simulink model "TC_SIM_FAST"  (R2025b)
settings: Solver=VariableStepAuto  StartTime=0.0  StopTime=10  RelTol=1e-6
values from neighbouring files (symbols this model uses):
  A = 1    [PARAMS.m]    (also in PARAMS_IDEAL_LAUNCH_TABLE.m; PID_TUNER.m)
  C = 16.56    [PARAMS.m]    (also in PARAMS_IDEAL_LAUNCH_TABLE.m; PID_TUNER.m; r20_18_drive_brake_processing_aaron_comparison.m = -1.75)
  Cd = 1    [PARAMS.m]    (also in PARAMS_IDEAL_LAUNCH_TABLE.m; PID_TUNER.m)
  cg_f = 0.734568    [PARAMS.m]    (also in PARAMS_IDEAL_LAUNCH_TABLE.m; PID_TUNER.m)
  Cl = 3.8    [PARAMS.m]    (also in PARAMS_IDEAL_LAUNCH_TABLE.m; PID_TUNER.m)
  Cp = 0.53    [PARAMS.m]    (also in PARAMS_IDEAL_LAUNCH_TABLE.m; PID_TUNER.m)
  D = 0    [PID_TUNER.m]
  Drive_Train = 0.89    [PARAMS.m]    (also in PARAMS_IDEAL_LAUNCH_TABLE.m; PID_TUNER.m)
  End_Blend = 8.0    (= 8)    [PARAMS.m]    (also in PARAMS_IDEAL_LAUNCH_TABLE.m; PID_TUNER.m)
  fd = 4.5    [PARAMS.m]    (also in PARAMS_IDEAL_LAUNCH_TABLE.m; PID_TUNER.m)
  gravity = 9.80665    [PARAMS.m]    (also in PARAMS_IDEAL_LAUNCH_TABLE.m; PID_TUNER.m)
  Grip_Fact = 1.0    (= 1)    [PARAMS.m]    (also in PARAMS_IDEAL_LAUNCH_TABLE.m; PID_TUNER.m)
  Grip_Influence = 1.2    [PARAMS.m]    (also in PARAMS_IDEAL_LAUNCH_TABLE.m; PID_TUNER.m)
  h_cg = 0.25273    [PARAMS.m]    (also in PARAMS_IDEAL_LAUNCH_TABLE.m; PID_TUNER.m)
  J_Motor = 0.34661    [PARAMS.m]    (also in PARAMS_IDEAL_LAUNCH_TABLE.m; PID_TUNER.m)
  J_Wheel = 0.16490    (= 0.1649)    [PARAMS.m]    (also in PARAMS_IDEAL_LAUNCH_TABLE.m; PID_TUNER.m)
  K = 5105.49    [PARAMS.m]    (also in PARAMS_IDEAL_LAUNCH_TABLE.m; PID_TUNER.m)
  Mv = 285.763    [PARAMS.m]    (also in PARAMS_IDEAL_LAUNCH_TABLE.m; PID_TUNER.m)
  r = 0.203    [PARAMS.m]    (also in PARAMS_IDEAL_LAUNCH_TABLE.m; PID_TUNER.m)
  rho = 1.225    [PARAMS.m]    (also in PARAMS_IDEAL_LAUNCH_TABLE.m; PID_TUNER.m)
  Slip_Target = 0.13    [PARAMS.m]    (also in PARAMS_IDEAL_LAUNCH_TABLE.m; PID_TUNER.m)
  Start_Blend = 3.0    (= 3)    [PARAMS.m]    (also in PARAMS_IDEAL_LAUNCH_TABLE.m; PID_TUNER.m)
  tau_motor = 0.03    [PARAMS.m]    (also in PARAMS_IDEAL_LAUNCH_TABLE.m; PID_TUNER.m = 0.02)
  Throttle_pts = double(launchCmd)/1000    [PARAMS.m]    (also in PARAMS_IDEAL_LAUNCH_TABLE.m = double(launchCmd)/1000.0; PID_TUNER.m = [0.000, 0.364, 0.600, 0.830, 0.903, 0.920, 0.917, 0.903, 0.9; THROTTLE_LOOKUP_GENERATOR.m = [1.000, 1.000, 1.000, 1.000, 1.000, 1.000, 1.000, 1.000, 1.0)
  Time_pts = double(launchTimeMs)/1000    [PARAMS.m]    (also in PARAMS_IDEAL_LAUNCH_TABLE.m = double(launchTimeMs)/1000.0; PID_TUNER.m = [0.000, 0.016, 0.033, 0.051, 0.072, 0.096, 0.121, 0.148, 0.1; THROTTLE_LOOKUP_GENERATOR.m = [0.000, 0.016, 0.033, 0.051, 0.072, 0.096, 0.121, 0.148, 0.1)
  Ts = 0.01    [PID_TUNER.m]
  W = 1.53035    [PARAMS.m]    (also in PARAMS_IDEAL_LAUNCH_TABLE.m; PID_TUNER.m)
undefined symbols (not defined in the file or in its folder): dspblkCoreblockFVToolHelper, gcbh, I, P
settings Model: Creator=jacks  LastModifiedBy=jacks
settings SolverCC: ZeroCrossAlgorithm=Adaptive
settings HardwareCC: ProdHWDeviceType=AMD->x86-64 (Windows64)

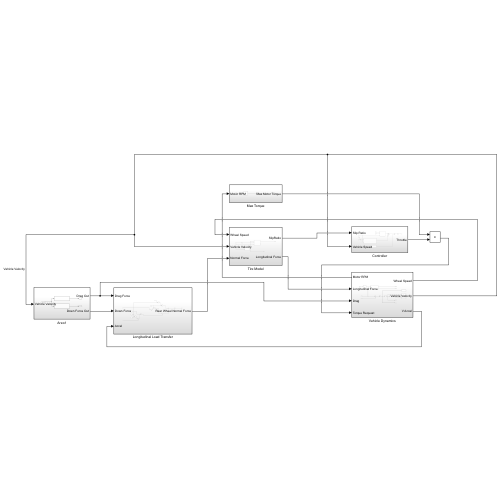
[thumbnail: Simulink's stored preview of the top-level diagram]
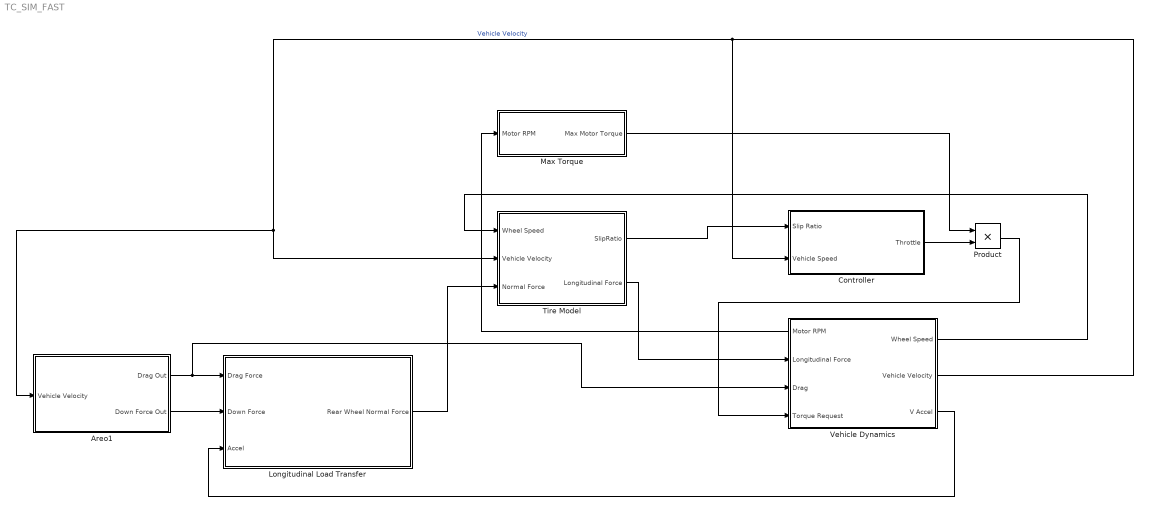
== system TC_SIM_FAST ==
  Areo1 : Subsystem
  Controller : Subsystem
  Longitudinal Load Transfer : Subsystem
  Max Torque : Subsystem
  Product : Product
  Tire Model : Subsystem
  Vehicle Dynamics : Subsystem
      settings: PortSchema="{\"entries\":[{\"content\":{\"sides\":[{\"content\":{\"connectorIds\":[\"Out4\",\"In1\",\"In2\",\"In3\"]},\"type\":\"ConnectorPlacement.EquallySpacedRectSide\",\"uuid\":\"581df02b-a84f-47c8-a58e-bf6c459b1ed9\"},{\"content\":{\"connectorIds\":[\"Out1\",\"Out2\",\"Out3\"],\"side\":\"RIGHT\"},\"type\":\"ConnectorPlacement.EquallySpacedRectSide\",\"uuid\":\"b0aa9a3f-0241-40f7-a584-ab2415552723\"},{\"content\":{\"side\":\"TOP\"},\"type\":\"ConnectorPlacement.EquallySpacedRectSide\",\"uuid\":\"02294242-5d66-4b6c-8820-16b0cf15de35\"}]},\"type\":\"ConnectorPlacement.EquallySpacedConnector\",\"uuid\":\"c4512b92-6de7-465b-80c8-945d7e9b8206\"}],\"packageUris\":[\"http://schema.mathworks.com/mf0/Connector/R2020b\"],\"version\":\"1.0\"}"
  wires:
  Vehicle Dynamics/2(Vehicle Velocity) -> Controller/2(Vehicle Speed), Tire Model/2(Vehicle Velocity), Areo1/1(Vehicle Velocity)  "Vehicle Velocity"
  Areo1/2(Down Force Out) -> Longitudinal Load Transfer/2(Down Force)
  Areo1/1(Drag Out) -> Longitudinal Load Transfer/1(Drag Force), Vehicle Dynamics/2(Drag)
  Vehicle Dynamics/3(V Accel) -> Longitudinal Load Transfer/3(Accel)
  Longitudinal Load Transfer/1(Rear Wheel Normal Force) -> Tire Model/3("Normal Force ")
  Tire Model/2(Longitudinal Force) -> Vehicle Dynamics/1(Longitudinal Force)
  Vehicle Dynamics/1(Wheel Speed) -> Tire Model/1(Wheel Speed)
  Vehicle Dynamics/4(Motor RPM) -> Max Torque/1(Motor RPM)
  Tire Model/1(SlipRatio) -> Controller/1(Slip Ratio)
  Max Torque/1(Max Motor Torque) -> Product/1
  Controller/1(Throttle) -> Product/2
  Product/1 -> Vehicle Dynamics/3(Torque Request)

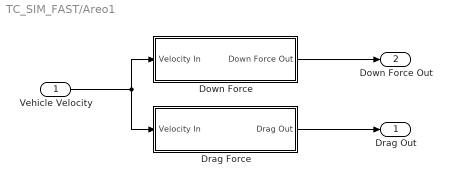
== system TC_SIM_FAST/Areo1 ==
  Vehicle Velocity : Inport
  Down Force : Subsystem
  Drag Force : Subsystem
  Drag Out : Outport
  Down Force Out : Outport  Port=2
  wires:
  Down Force/1(Down Force Out) -> Down Force Out/1
  Vehicle Velocity/1 -> Drag Force/1(Velocity In), Down Force/1(Velocity In)
  Drag Force/1(Drag Out) -> Drag Out/1

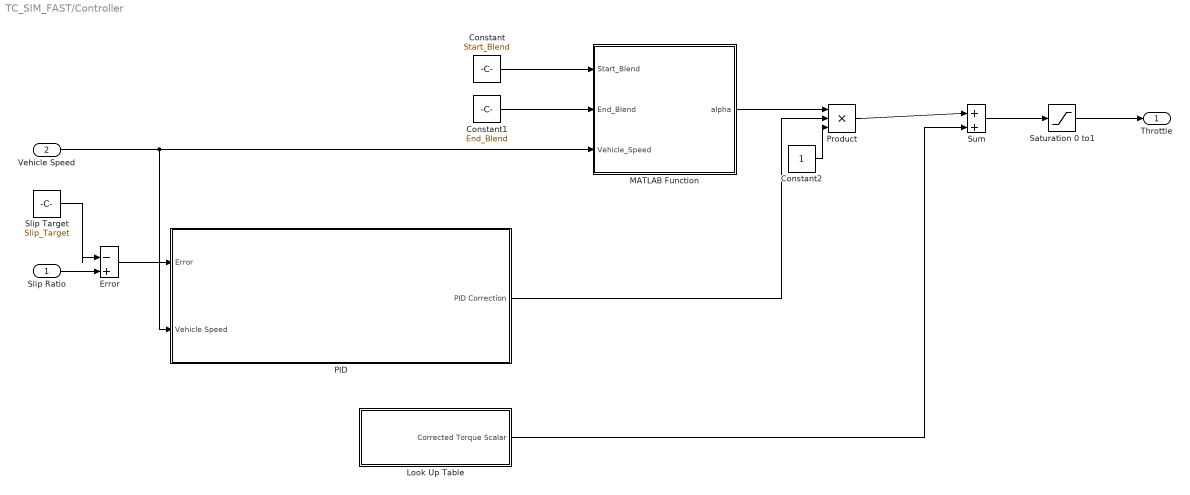
== system TC_SIM_FAST/Controller ==
  Slip Ratio : Inport
  Vehicle Speed : Inport  Port=2
  Constant : Constant  Value=Start_Blend
  Constant1 : Constant  Value=End_Blend
  Constant2 : Constant
  Error : Sum  Inputs=|-+
  Look Up Table : Subsystem
  MATLAB Function : MATLAB Function  TreatAsAtomicUnit=on
  PID : Subsystem
  Product : Product  Inputs=3
  Saturation 0 to1 : Saturate  UpperLimit=1  LowerLimit=0
  Slip Target : Constant  Value=Slip_Target
  Sum : Sum  Inputs=|++
  Throttle : Outport
  wires:
  Slip Target/1 -> Error/1
  Error/1 -> PID/1(Error)
  Vehicle Speed/1 -> PID/2(Vehicle Speed), MATLAB Function/3(Vehicle_Speed)
  Look Up Table/1(Corrected Torque Scalar) -> Sum/2
  Sum/1 -> Saturation 0 to1/1
  Slip Ratio/1 -> Error/2
  Saturation 0 to1/1 -> Throttle/1
  Constant1/1 -> MATLAB Function/2(End_Blend)
  Constant/1 -> MATLAB Function/1(Start_Blend)
  MATLAB Function/1(alpha) -> Product/1
  PID/1(PID Correction) -> Product/2
  Product/1 -> Sum/1
  Constant2/1 -> Product/3

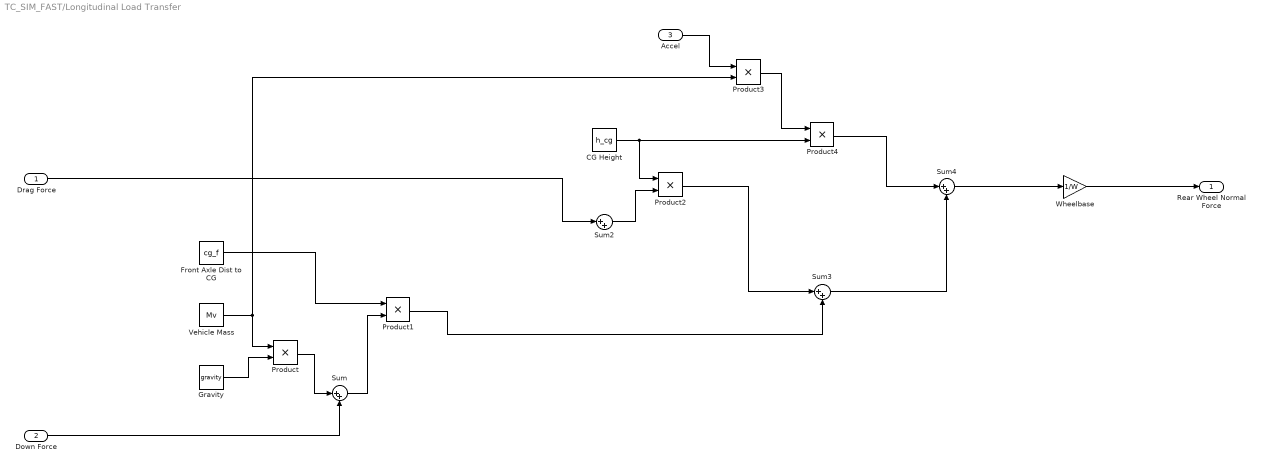
== system TC_SIM_FAST/Longitudinal Load Transfer ==
  Drag Force : Inport
  Down Force : Inport  Port=2
  Accel : Inport  Port=3
  CG Height : Constant  Value=h_cg
  Front Axle Dist to CG : Constant  Value=cg_f
  Gravity : Constant  Value=gravity
  Product{,1..4} (5 alike) : Product
  Sum{,2..4} (4 alike) : Sum  Inputs=|++
  Vehicle Mass : Constant  Value=Mv
  Wheelbase : Gain  Gain=1/W
  Rear Wheel Normal Force : Outport
  wires:
  Vehicle Mass/1 -> Product3/2, Product/1
  Gravity/1 -> Product/2
  Down Force/1 -> Sum/2
  Product/1 -> Sum/1
  Sum/1 -> Product1/2
  Front Axle Dist to CG/1 -> Product1/1
  Drag Force/1 -> Sum2/1
  CG Height/1 -> Product4/2, Product2/1
  Sum2/1 -> Product2/2
  Accel/1 -> Product3/1
  Product3/1 -> Product4/1
  Product2/1 -> Sum3/1
  Product1/1 -> Sum3/2
  Product4/1 -> Sum4/1
  Sum3/1 -> Sum4/2
  Sum4/1 -> Wheelbase/1
  Wheelbase/1 -> Rear Wheel Normal Force/1

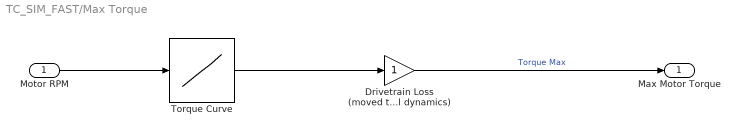
== system TC_SIM_FAST/Max Torque ==
  Motor RPM : Inport
  "Drivetrain Loss (moved to wheel dynamics) " : Gain
  Torque Curve : Lookup_n-D  NumberOfTableDimensions=1  BreakpointsForDimension1=[0,100,200,300,400,500,600,700,800,900,1000,1100,1200,1300,1400,1500,1600,1700,1800,1900,2000,2100,2200,2300,2400,2500,2600,2700,2800,2900,3000,3100,3200,3300,3400,3500,3600,3700,3800,3820,3900,4000,4100,4200,4300,4400,4500,4600,4700,4800,4900,5000,5100,5200,5300,5400,5500,5600,5700,5800,5900,6000,6100,6200,6300,6400,6500,6600,6700,6800,6900,7000]  Table=[140,142,144,146,148,150,150,150,150,150,150,150,150,150,150,150,150,150,150,150,150,150,150,150,150,150,150,150,150,150,150,150,150,150,150,150,150,150,150,150,150,150,150,150,150,150,150,150,150,149.2,146.2,143.2,140.4,137.7,135.1,132.6,130.2,127.9,125.6,123.5,121.4,119.4,117.4,115.5,113.7,111.9,110.2,108.5,106.9,105.3,103.8,102.3]  InternalRulePriority=Speed  RndMeth=Simplest
  Max Motor Torque : Outport
  wires:
  Torque Curve/1 -> "Drivetrain Loss (moved to wheel dynamics) "/1
  "Drivetrain Loss (moved to wheel dynamics) "/1 -> Max Motor Torque/1  "Torque Max"
  Motor RPM/1 -> Torque Curve/1

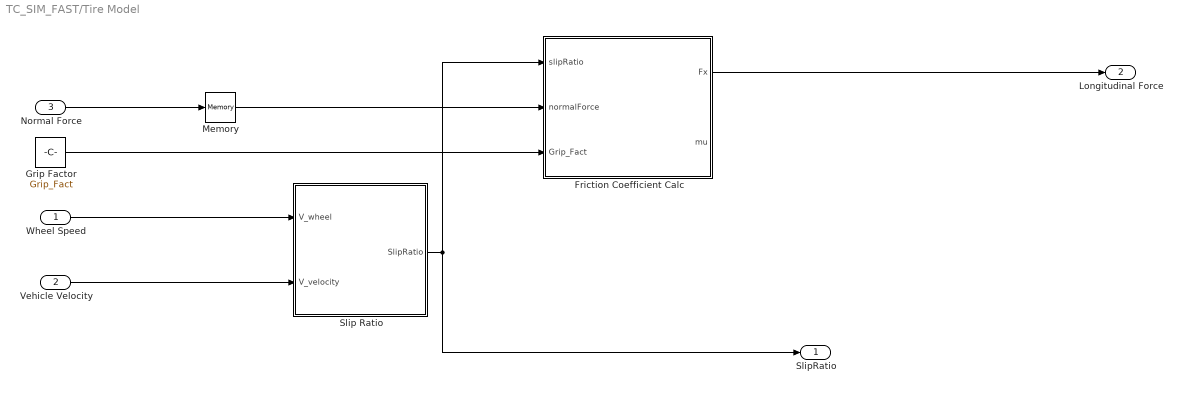
== system TC_SIM_FAST/Tire Model ==
  Wheel Speed : Inport
  Vehicle Velocity : Inport  Port=2
  "Normal Force " : Inport  Port=3
  Friction Coefficient Calc : MATLAB Function  TreatAsAtomicUnit=on
  Grip Factor : Constant  Value=Grip_Fact
  Memory : Memory
  Slip Ratio : MATLAB Function  TreatAsAtomicUnit=on
  SlipRatio : Outport
  Longitudinal Force : Outport  Port=2
  wires:
  Slip Ratio/1(SlipRatio) -> SlipRatio/1, Friction Coefficient Calc/1(slipRatio)
  Vehicle Velocity/1 -> Slip Ratio/2(V_velocity)
  Wheel Speed/1 -> Slip Ratio/1(V_wheel)
  "Normal Force "/1 -> Memory/1
  Friction Coefficient Calc/1(Fx) -> Longitudinal Force/1
  Memory/1 -> Friction Coefficient Calc/2(normalForce)
  Grip Factor/1 -> Friction Coefficient Calc/3(Grip_Fact)

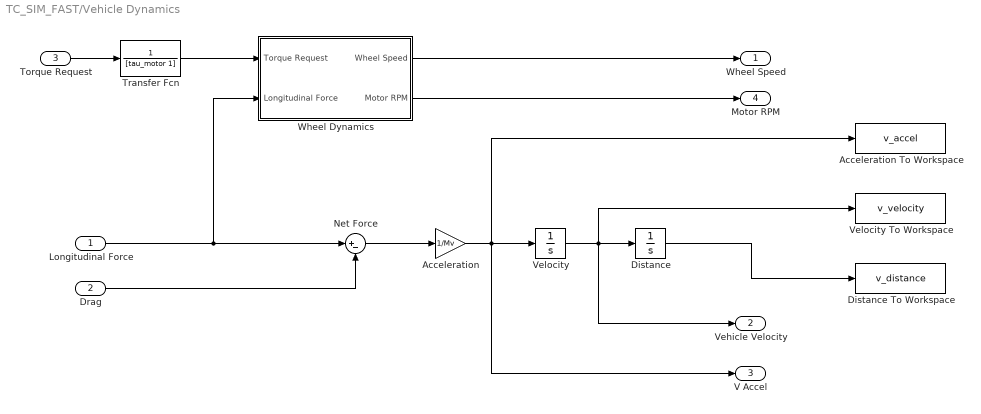
== system TC_SIM_FAST/Vehicle Dynamics ==
  Longitudinal Force : Inport
  Drag : Inport  Port=2
  Torque Request : Inport  Port=3
  Acceleration : Gain  Gain=1/Mv
  Acceleration To Workspace : ToWorkspace  VariableName=v_accel  SaveFormat=Timeseries  SampleTime=-1
  Distance : Integrator
  Distance To Workspace : ToWorkspace  VariableName=v_distance  SaveFormat=Timeseries  SampleTime=-1
  Net Force : Sum  Inputs=|+-
  Transfer Fcn : TransferFcn  Denominator=[tau_motor 1]
  "Velocity " : Integrator  InitialCondition=0.0001
  Velocity To Workspace : ToWorkspace  VariableName=v_velocity  SaveFormat=Timeseries  SampleTime=-1
  Wheel Dynamics : Subsystem
  Wheel Speed : Outport
  Vehicle Velocity : Outport  Port=2
  V Accel : Outport  Port=3
  Motor RPM : Outport  Port=4
  wires:
  "Velocity "/1 -> Vehicle Velocity/1, Velocity To Workspace/1, Distance/1
  Acceleration/1 -> V Accel/1, "Velocity "/1, Acceleration To Workspace/1
  Distance/1 -> Distance To Workspace/1
  Drag/1 -> Net Force/2
  Net Force/1 -> Acceleration/1
  Longitudinal Force/1 -> Net Force/1, Wheel Dynamics/2(Longitudinal Force)
  Wheel Dynamics/2(Motor RPM) -> Motor RPM/1
  Wheel Dynamics/1(Wheel Speed) -> Wheel Speed/1
  Torque Request/1 -> Transfer Fcn/1
  Transfer Fcn/1 -> Wheel Dynamics/1(Torque Request)

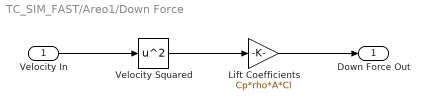
== system TC_SIM_FAST/Areo1/Down Force ==
  Velocity In : Inport
  Lift Coefficients : Gain  Gain=Cp*rho*A*Cl
  Velocity Squared : Math  Operator=square
  Down Force Out : Outport
  wires:
  Velocity Squared/1 -> Lift Coefficients/1
  Lift Coefficients/1 -> Down Force Out/1
  Velocity In/1 -> Velocity Squared/1

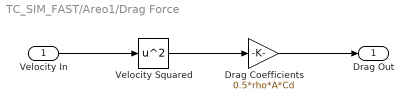
== system TC_SIM_FAST/Areo1/Drag Force ==
  Velocity In : Inport
  Drag Coefficients : Gain  Gain=0.5*rho*A*Cd
  Velocity Squared : Math  Operator=square
  Drag Out : Outport
  wires:
  Velocity In/1 -> Velocity Squared/1
  Velocity Squared/1 -> Drag Coefficients/1
  Drag Coefficients/1 -> Drag Out/1

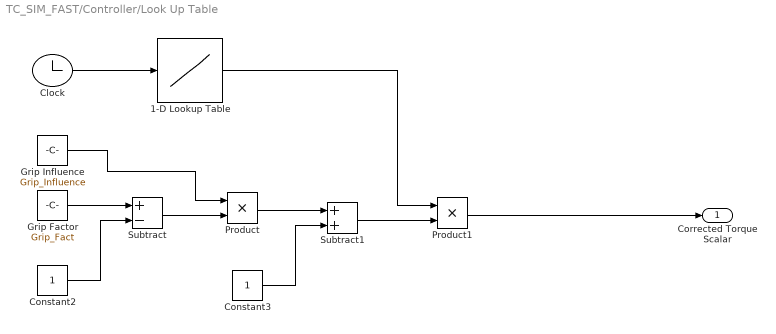
== system TC_SIM_FAST/Controller/Look Up Table ==
  1-D Lookup Table : Lookup_n-D  NumberOfTableDimensions=1  BreakpointsForDimension1=Time_pts  Table=Throttle_pts  InternalRulePriority=Speed  RndMeth=Simplest
  Clock : Clock
  Constant2 : Constant
  Constant3 : Constant
  Grip Factor : Constant  Value=Grip_Fact
  Grip Influence : Constant  Value=Grip_Influence
  Product : Product
  Product1 : Product
  Subtract : Sum  Inputs=+-
  Subtract1 : Sum
  Corrected Torque Scalar : Outport
  wires:
  Grip Factor/1 -> Subtract/1
  Constant2/1 -> Subtract/2
  Grip Influence/1 -> Product/1
  Subtract/1 -> Product/2
  Constant3/1 -> Subtract1/2
  Product/1 -> Subtract1/1
  Subtract1/1 -> Product1/2
  Product1/1 -> Corrected Torque Scalar/1
  Clock/1 -> 1-D Lookup Table/1
  1-D Lookup Table/1 -> Product1/1

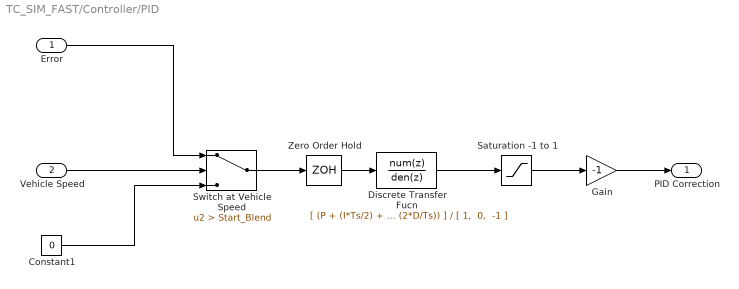
== system TC_SIM_FAST/Controller/PID ==
  Error : Inport
  Vehicle Speed : Inport  Port=2
  Constant1 : Constant  Value=0
  Discrete Transfer Fucn : DiscreteTransferFcn  LoadFcn=dspblkCoreblockFVToolHelper(gcbh,'load');  Numerator="[ (P + (I*Ts/2) + (2*D/Ts)),  ((I*Ts) - (4*D/Ts)),  (-P + (I*Ts/2) + (2*D/Ts)) ]"  Denominator="[ 1,  0,  -1 ]"
      settings: CopyFcn=dspblkCoreblockFVToolHelper(gcbh,'copy');  DeleteFcn=dspblkCoreblockFVToolHelper(gcbh,'close');  ModelCloseFcn=dspblkCoreblockFVToolHelper(gcbh,'close');  PreSaveFcn=dspblkCoreblockFVToolHelper(gcbh,'presave');  PostSaveFcn=dspblkCoreblockFVToolHelper(gcbh,'postsave');  CloseFcn=dspblkCoreblockFVToolHelper(gcbh,'close');
  Gain : Gain  Gain=-1
  Saturation -1 to 1 : Saturate  UpperLimit=1  LowerLimit=-1
  Switch at Vehicle Speed : Switch  Criteria=u2 > Threshold  Threshold=Start_Blend  SaturateOnIntegerOverflow=off  InputSameDT=off
  Zero Order Hold : ZeroOrderHold  SampleTime=Ts
  PID Correction : Outport
  wires:
  Switch at Vehicle Speed/1 -> Zero Order Hold/1
  Zero Order Hold/1 -> Discrete Transfer Fucn/1
  Error/1 -> Switch at Vehicle Speed/1
  Saturation -1 to 1/1 -> Gain/1
  Vehicle Speed/1 -> Switch at Vehicle Speed/2
  Constant1/1 -> Switch at Vehicle Speed/3
  Discrete Transfer Fucn/1 -> Saturation -1 to 1/1
  Gain/1 -> PID Correction/1

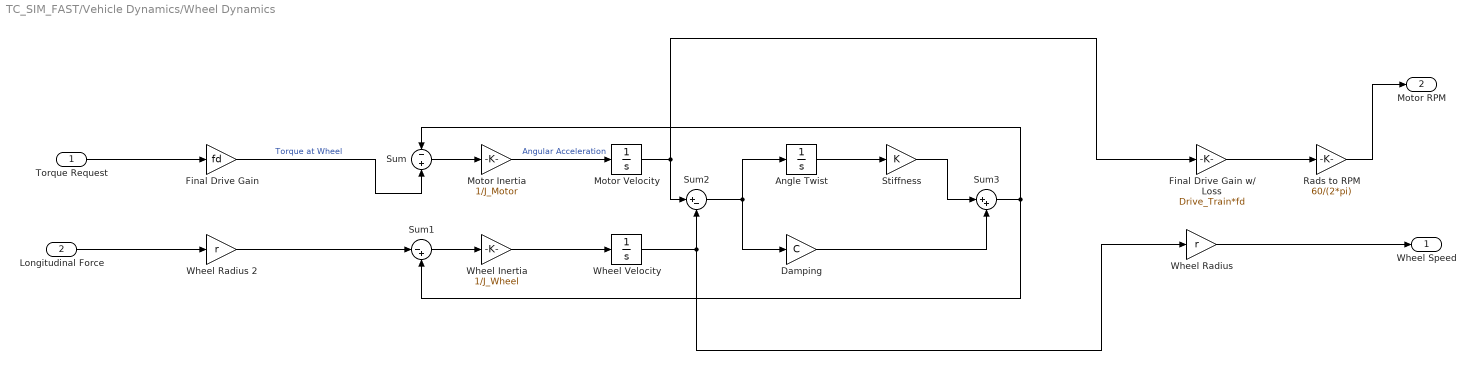
== system TC_SIM_FAST/Vehicle Dynamics/Wheel Dynamics ==
  Torque Request : Inport
  Longitudinal Force : Inport  Port=2
  Angle Twist : Integrator
  Damping : Gain  Gain=C
  Final Drive Gain : Gain  Gain=fd
  Final Drive Gain w/ Loss : Gain  Gain=Drive_Train*fd
  Motor Inertia : Gain  Gain=1/J_Motor
  Motor Velocity : Integrator
  Rads to RPM : Gain  Gain=60/(2*pi)
  Stiffness : Gain  Gain=K
  Sum : Sum  Inputs=-+
  Sum1 : Sum  Inputs=|-+
  Sum2 : Sum  Inputs=|+-
  Sum3 : Sum  Inputs=|++
  Wheel Inertia : Gain  Gain=1/J_Wheel
  Wheel Radius : Gain  Gain=r
  Wheel Radius 2 : Gain  Gain=r
  Wheel Velocity : Integrator
  Wheel Speed : Outport
  Motor RPM : Outport  Port=2
  wires:
  Torque Request/1 -> Final Drive Gain/1
  Longitudinal Force/1 -> Wheel Radius 2/1
  Wheel Radius/1 -> Wheel Speed/1
  Final Drive Gain w/ Loss/1 -> Rads to RPM/1
  Rads to RPM/1 -> Motor RPM/1
  Wheel Velocity/1 -> Sum2/2, Wheel Radius/1
  Sum/1 -> Motor Inertia/1
  Motor Inertia/1 -> Motor Velocity/1  "Angular Acceleration"
  Wheel Radius 2/1 -> Sum1/1
  Sum1/1 -> Wheel Inertia/1
  Wheel Inertia/1 -> Wheel Velocity/1
  Motor Velocity/1 -> Final Drive Gain w/ Loss/1, Sum2/1
  Sum2/1 -> Damping/1, Angle Twist/1
  Stiffness/1 -> Sum3/1
  Damping/1 -> Sum3/2
  Angle Twist/1 -> Stiffness/1
  Sum3/1 -> Sum/1, Sum1/2
  Final Drive Gain/1 -> Sum/2  "Torque at Wheel"

== matlab function TC_SIM_FAST/Tire Model/Friction Coefficient Calc ==
  data: slipRatio input; Fx output; normalForce input; mu output; Grip_Fact input
function [Fx, mu] = calculatePacejkaFx(slipRatio, normalForce, Grip_Fact)

% normalForce is total rear axle normal force [N]
% Fx output is total rear axle longitudinal force [N]

B  = coder.const(10.4);
C  = coder.const(1.58);
D1 = coder.const(3.02);
D2 = coder.const(0.0008 / 4.448221615); % convert from per lbf to per N

Fz_rear = max(normalForce, 0);
Fz_tire = Fz_rear/2;

mu = (D1 - D2*Fz_tire) * Grip_Fact;
mu = max(mu, 0);

Fx_tire = mu * Fz_tire * sin(C * atan(B * slipRatio));

% Two driven rear tires
Fx = 2*Fx_tire;

end

== matlab function TC_SIM_FAST/Tire Model/Slip Ratio ==
  data: V_wheel input; SlipRatio output; V_velocity input
function SlipRatio = compute_slip(V_wheel, V_velocity)
    eps_val = cast(0.5, 'like', V_velocity);   
    den = max(max(abs(V_velocity), abs(V_wheel)), eps_val);  
    SlipRatio = (V_wheel - V_velocity) / den;
end

== matlab function TC_SIM_FAST/Controller/MATLAB Function ==
  data: Start_Blend input; alpha output; End_Blend input; Vehicle_Speed input
function alpha = blend_alpha(Start_Blend, End_Blend, Vehicle_Speed)

% Smoothly blends from 0 to 1 based on vehicle speed

    % Prevent divide-by-zero or bad inputs
    if End_Blend <= Start_Blend
        if Vehicle_Speed >= End_Blend
            alpha = 1;
        else
            alpha = 0;
        end
        return;
    end

    % Linear blend
    alpha = (Vehicle_Speed - Start_Blend) / (End_Blend - Start_Blend);

    % Clamp to 0 to 1
    if alpha < 0
        alpha = 0;
    elseif alpha > 1
        alpha = 1;
    end

    % Smoothstep shaping
    alpha = alpha * alpha * (3 - 2 * alpha);
end
